simulink model "starshotsimv5"  (R2023a)
settings: Solver=FixedStepAuto  StartTime=0.0  StopTime=350000  FixedStep=0.01  MaxStep=4.0  MinStep=.001  RelTol=1e-6
undefined symbols (not defined in the file): B0, DiscIntNeverNeededParam, G, M_Earth, q0, R_Earth, starshot
libraries: dspmathops x3, vrlib x2, simulink x2, sharedtransform x1
(part 2 of 2)

== system starshotsimv5/StarshotACS/Orientation controller/sign_function1 ==
  omega : Inport
  Constant10 : Constant  Value=-1
  Constant9 : Constant
  Selector : Selector  InputPortWidth=3  IndexOptions=Index vector (dialog)  Indices=[3]  OutputSizes=1
  Switch1 : Switch  ZeroCross=off  SaturateOnIntegerOverflow=off  InputSameDT=off
  sign(omega_z) : Outport
  wires:
  Constant9/1 -> Switch1/1
  Constant10/1 -> Switch1/3
  Switch1/1 -> sign(omega_z)/1
  Selector/1 -> Switch1/2
  omega/1 -> Selector/1

== system starshotsimv5/Plant_OG/   /Normalized quat/Modulo1 ==
  q : Inport
  Demux2 : Demux
      settings: DisplayOption=none
  Math Function{1..4} (4 alike) : Math  Operator=square  SignedPower=on
  Math Function5 : Math  Operator=sqrt  SignedPower=on
  Sum5 : Sum  Inputs=|++++  SaturateOnIntegerOverflow=on
  Module q : Outport
  wires:
  q/1 -> Demux2/1
  Math Function5/1 -> Module q/1
  Sum5/1 -> Math Function5/1
  Math Function4/1 -> Sum5/3
  Math Function3/1 -> Sum5/2
  Math Function1/1 -> Sum5/1
  Demux2/3 -> Math Function4/1
  Demux2/2 -> Math Function3/1
  Demux2/1 -> Math Function1/1
  Demux2/4 -> Math Function2/1
  Math Function2/1 -> Sum5/4

== system starshotsimv5/StarshotACS/Orientation controller/Subsystem1/Norm4 ==
  v : Inport
  Dot Product6 : DotProduct  OutDataTypeStr=Inherit: Inherit via internal rule
  Sqrt4 : Sqrt
  norm(v) : Outport
  wires:
  v/1 -> Dot Product6/1, Dot Product6/2
  Dot Product6/1 -> Sqrt4/1
  Sqrt4/1 -> norm(v)/1

== system starshotsimv5/StarshotACS/Orientation controller/Subsystem1/Norm5 ==
  v : Inport
  Dot Product6 : DotProduct  OutDataTypeStr=Inherit: Inherit via internal rule
  Sqrt4 : Sqrt
  norm(v) : Outport
  wires:
  v/1 -> Dot Product6/1, Dot Product6/2
  Dot Product6/1 -> Sqrt4/1
  Sqrt4/1 -> norm(v)/1
